simulink model "psb3phpll"  (Simulink 6.0)
settings: Solver=FixedStepDiscrete  SolverMode=SingleTasking  StartTime=0.0  StopTime=3.5  RelTol=1e-3  AbsTol=1e-2
InitFcn:
  | powericon('psbinitsys',bdroot);
libraries: powerlib2 x6, powerlib_extras x3
settings Model: Creator=sybille  LastModifiedBy=batserve  ExtModeTrigMode=oneshot  ExtModeArmWhenConnect=off  ExtModeAutoUpdateStatusClock=off  ProdHWDeviceType=Specified
settings DataIOCC: Decimation=10  LimitDataPoints=off  SaveFinalState=on  SaveOutput=off  SignalLoggingName=sigsOut
settings OptimizationCC: BlockReduction=off  BooleanDataType=off
settings DebuggingCC: CheckExecutionContextPreStartOutputMsg=on  CheckExecutionContextRuntimeOutputMsg=on  SolverPrmCheckMsg=none  UnconnectedInputMsg=none  UnconnectedOutputMsg=none
settings HardwareCC: ProdBitPerShort=32  ProdBitPerInt=16  ProdHWDeviceType=Specified  TargetUnknown=on
settings RTWCC: TemplateMakefile=grt_vc.tmf

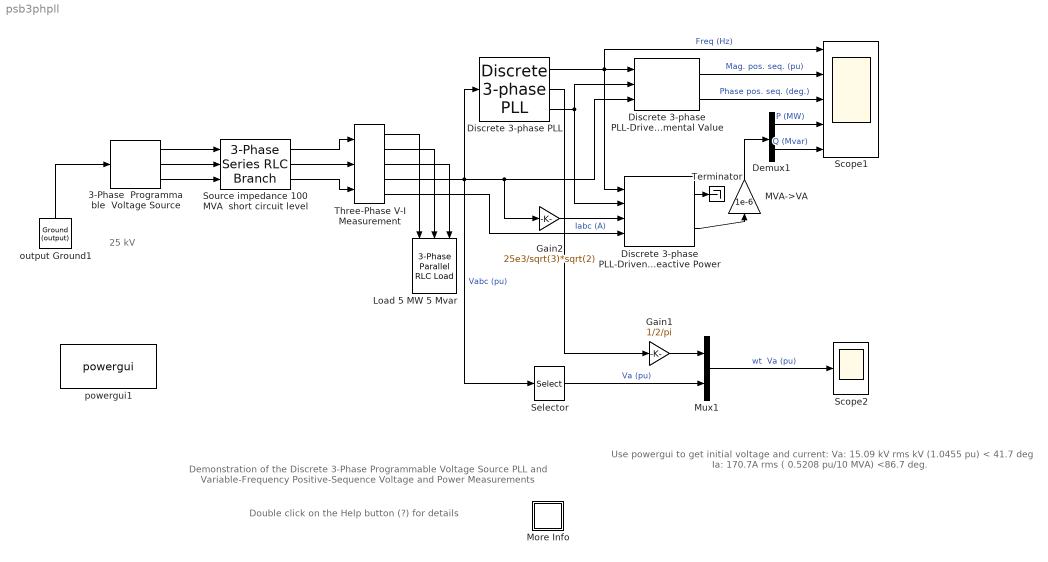
== system psb3phpll ==
  note: Demonstration of the Discrete 3-Phase Programmable Voltage Source
      | PLL and Variable-Frequency Positive-Sequence Voltage and Power Measurements
  note: Double click on the Help button (?) for details
  note: Use powergui to get initial voltage and current:
      | Va: 15.09 kV rms  kV (1.0455 pu) < 41.7 deg
      | Ia: 170.7A rms ( 0.5208 pu/10 MVA) <86.7 deg.
  note: 25 kV
  3-Phase  Programmable  Voltage Source : powerlib2/Electrical Sources/3-Phase  Programmable  Voltage Source  Par_Vps_LLrms="[25e3  45 60]"  VariationEntity=Frequency  VariationType=Modulation  VariationStep=-0.5  VariationRate=10  VariationMag=3  VariationFreq=0.4  Par_Timing_Variation=[0.5 3.0]  SinglePhase=off  Yampli=[1 0.8 1.2 1.0]  Xtime=[0 0.1 0.15 0.2]  HarmonicGeneration=off  Par_HarmoA_pu=[3 0.2 -25 0]  Par_HarmoB_pu="[2 0.15  35 2]"  Par_Timing_Harmo="[0.05  3]"
  Demux1 : Demux  Outputs=2
  Discrete 3-phase PLL : powerlib_extras/Discrete  Control Blocks/Discrete 3-phase PLL  Fmin=45  Par_Init=[41.7 60]  ParK=[60 1400]  Ts=50e-6
  Discrete 3-phase PLL-Driven Positive-Sequence Fundamental Value : powerlib_extras/Discrete Measurements/Discrete 3-phase PLL-Driven Positive-Sequence Fundamental Value  Finit=60  Fmin=45  Par_Init=[1.0455 41.7]  Ts=50e-6
  Discrete 3-phase PLL-Driven  Positive-Sequence Active & Reactive Power : powerlib_extras/Discrete Measurements/Discrete 3-phase PLL-Driven  Positive-Sequence Active & Reactive Power  Finit=60  Fmin=45  Par_Vinit=[15.09e3*sqrt(2) 41.7]  Par_Iinit=[170.7*sqrt(2) 86.7]  Ts=50e-6
  Gain1 : Gain  Gain=1/2/pi  SaturateOnIntegerOverflow=on
  Gain2 : Gain  Gain=25e3/sqrt(3)*sqrt(2)  SaturateOnIntegerOverflow=on
  Load 5 MW 5 Mvar : powerlib2/Elements/3-Phase Parallel RLC Load  Orientation=down  Vpp=25e3  fn=60  P3=5e6  QL3=0  QC3=5e6
  MVA->VA : Gain  Orientation=up  Gain=1e-6  SaturateOnIntegerOverflow=on
  More Info : Subsystem
      mask Display: disp('?')
  Mux1 : Mux  Inputs=2
  Scope1 : Scope  NumInputPorts=5
      settings: TimeRange=3.5  YMin=56~1.04~-2~5.41~-5.800000000000001  YMax=64~1.051~2~5.529999999999999~-5.1  DataFormat=Array  SampleInput=on
  Scope2 : Scope
      settings: TimeRange=0.05  YMin=-1.1  YMax=1.1  DataFormat=Array  SampleInput=on
  Selector : Selector  InputPortWidth=3
  Source impedance 100 MVA  short circuit level : powerlib2/Elements/3-Phase Series RLC Branch   R=25^2/100/10  L=25^2/100/377  C=inf
  Terminator : Terminator
  Three-Phase V-I Measurement : powerlib2/Measurements/Three-Phase V-I Measurement  Tag=PoWeRsYsTeMmEaSuReMeNt  VChoice=phase-to-ground  ualv=off  labelV=V1  Vpu=on  Vbase=25e3  IChoice=yes  ualc=off  labelC=I1  Ppu=off  Pbase=10e6  OutputType=Magnitude  PhasorSimulation=off  PSBequivalent=1  PSBOutputType=11100
  output Ground1 : powerlib2/Connectors/Ground (output)  Tag=PoWeRsYsTeMbLoCk  Orientation=up  PSBOutputType=1
  powergui1 : powerlib2/powergui  Frange=[0:2:500]  Ylog=off  Xlog=off  save=off  variable=ZData  ZoomFFT=on  StartTime=0.0  cycles=1  DisplayStyle=off  fundamental=60  FreqAxis=off  MaxFrequency=1000  frequencyindice=1  frequencyindicesteady=1  RmsSteady=2  display=off  Ts=50e-6  methode=off  frequency=60  echomessages=off
  wires:
  Source impedance 100 MVA  short circuit level/1 -> Three-Phase V-I Measurement/1
  Source impedance 100 MVA  short circuit level/2 -> Three-Phase V-I Measurement/2
  Source impedance 100 MVA  short circuit level/3 -> Three-Phase V-I Measurement/3
  Three-Phase V-I Measurement/1 -> Load 5 MW 5 Mvar/1
  Three-Phase V-I Measurement/2 -> Load 5 MW 5 Mvar/2
  Three-Phase V-I Measurement/3 -> Load 5 MW 5 Mvar/3
  Three-Phase V-I Measurement/4 -> Selector/1, Discrete 3-phase PLL/1, Discrete 3-phase PLL-Driven Positive-Sequence Fundamental Value/3, Gain2/1  "Vabc (pu)"
  Discrete 3-phase PLL/1 -> Discrete 3-phase PLL-Driven Positive-Sequence Fundamental Value/1, Scope1/1, Discrete 3-phase PLL-Driven  Positive-Sequence Active & Reactive Power/1  "Freq (Hz)"
  Discrete 3-phase PLL-Driven Positive-Sequence Fundamental Value/1 -> Scope1/2  "Mag. pos. seq. (pu)"
  Discrete 3-phase PLL-Driven Positive-Sequence Fundamental Value/2 -> Scope1/3  "Phase pos. seq. (deg.)"
  Gain1/1 -> Mux1/1
  Discrete 3-phase PLL/2 -> Gain1/1
  Mux1/1 -> Scope2/1  "wt  Va (pu)"
  Selector/1 -> Mux1/2  "Va (pu)"
  Discrete 3-phase PLL/3 -> Discrete 3-phase PLL-Driven Positive-Sequence Fundamental Value/2, Discrete 3-phase PLL-Driven  Positive-Sequence Active & Reactive Power/2
  Three-Phase V-I Measurement/5 -> Discrete 3-phase PLL-Driven  Positive-Sequence Active & Reactive Power/4  "Iabc (A)"
  Demux1/1 -> Scope1/4  "P (MW)"
  Demux1/2 -> Scope1/5  "Q (Mvar)"
  Gain2/1 -> Discrete 3-phase PLL-Driven  Positive-Sequence Active & Reactive Power/3
  Discrete 3-phase PLL-Driven  Positive-Sequence Active & Reactive Power/2 -> MVA->VA/1
  MVA->VA/1 -> Demux1/1
  Discrete 3-phase PLL-Driven  Positive-Sequence Active & Reactive Power/1 -> Terminator/1
  3-Phase  Programmable  Voltage Source/1 -> Source impedance 100 MVA  short circuit level/1
  3-Phase  Programmable  Voltage Source/2 -> Source impedance 100 MVA  short circuit level/2
  3-Phase  Programmable  Voltage Source/3 -> Source impedance 100 MVA  short circuit level/3
  output Ground1/1 -> 3-Phase  Programmable  Voltage Source/1

== system psb3phpll/More Info ==
  note: Circuit Description
  note: This demonstration ilustrates use of the 3-Phase Programmble Voltage Source,
      | PLL and Variable-Frequency Positive-Sequence Voltage and Power Measurement blocks
  note: A  25kV, 100 MVA short-circuit level,  equivalent network feeds a 5 MW, 5 Mvar capacitive load.
      | The internal voltage of the source is controlled by the Dicrete 3-Phase Programmable Voltage Source block.
      |
      | Open the programmable source dialog box and look at the parameters controlling the voltage and frequency.
      | A 60 Hz, positive-sequence of 1.0 pu, 45 degrees is specified.
      | At t = 0.5 s a sinusoidal modulation of the frequency (amplitude 3 Hz, frequency 0.4 Hz) is started.
      | The modulation stops at t =3 s so that a full cycle of modulation can be observed.
      |
      | The  Three-Phase V-I Measurement block is used to monitor the three load voltages and currents.
      | Open its dialog box and see how this block allows to output the three voltages and currents in p.u.
      |
      | The Discrete 3-Phase PLL block measures the frequency and generates a signal (wt output) locked on the variable frequency system voltage.
      | The PLL drives two  measurement blocks  taking into account the variable frequency: one block computing the  fundamental value
      | of the positive-sequence load voltage and another one computing the load active and reactive powers.
      | These two blocks and the PLL are initialized in order to start in steady state.
      | The PLL and and the two measurement  blocks are available respectively  in the Extras/Discrete Control Blocks and Extras/Discrete Measurements libraries.
      |
      | The whole system, (power network, PLL and measurement  blocks) is discretized at a 50 us sample time.
  note: Demonstration
  note: Select  Simulation/Start.
      |
      | Observe  on Scope1 block how the PLL tracks the  changing system frequency (trace 1).
      | As expected, the system frequency  varies between 57 Hz and 63 Hz with a maximum rate of change of 7.5 Hz/s.
      | Traces 2  and 3 show the variations of magnitude and phase of positive-sequence voltage as the frequency is changing.
      | Traces 4 and 5 show the variations of active and reactive powers.
      |
      | Observe on Scope2 that the (wt) ramp output of the PLL stays locked on zero crossings of phase A voltage.
  note: G. Sybille and P. Giroux (Hydro-Quebec)
